simulink model "Simulink_lab1"  (R2019a)
settings: Solver=VariableStepAuto  StartTime=0.0  StopTime=10.0  RelTol=1e-3
settings Model: Creator=T.S  LastModifiedBy=T.S

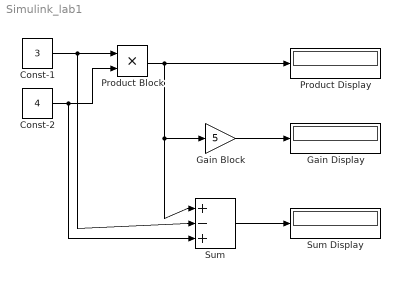
== system Simulink_lab1 ==
  Const-1 : Constant  Value=3
  Const-2 : Constant  Value=4
  "Gain Block " : Gain  Gain=5
  Gain Display : Display
  "Product Block " : Product
  Product Display : Display
  Sum : Sum  Inputs=|+-+
  Sum Display : Display
  wires:
  Const-2/1 -> Sum/3, "Product Block "/2
  Const-1/1 -> Sum/2, "Product Block "/1
  "Product Block "/1 -> Sum/1, "Gain Block "/1, Product Display/1
  "Gain Block "/1 -> Gain Display/1
  Sum/1 -> Sum Display/1
